simulink model "quadcopter_sim_1"  (R2023b)
settings: Solver=VariableStepAuto  StartTime=0.0  StopTime=10  RelTol=1e-3
libraries: simulink x2, mpclib x1, aerolibanimutils x1
settings Model: Creator=farhan  LastModifiedBy=farhan

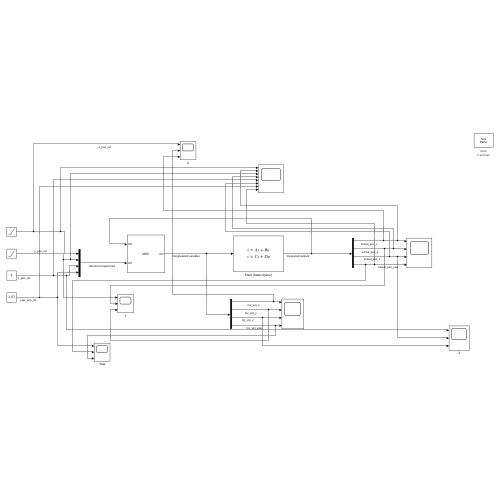
[thumbnail: Simulink's stored preview of the top-level diagram]
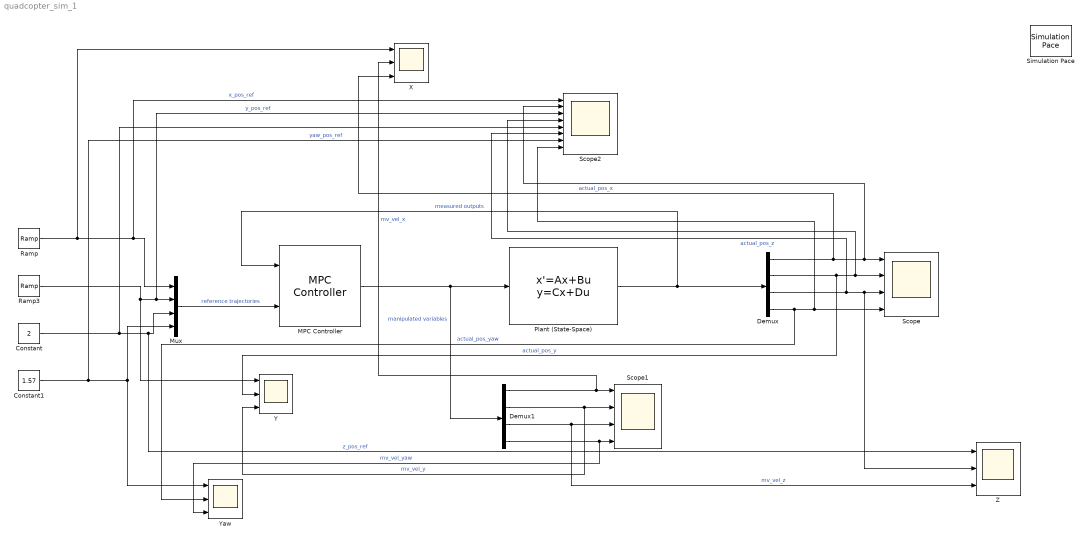
== system quadcopter_sim_1 ==
  Constant : Constant  Value=2
  Constant1 : Constant  Value=1.57
  Demux : Demux
  Demux1 : Demux
  MPC Controller : mpclib/MPC Controller  SCDEnableBlockLinearizationSpecification=on  mpcobj=mpc1  is_multiple=0  enable_value=0  return_u0=off  updateMPCinCallerWorkspace=on  md_inport=off  mv_inport=off  uref_inport=off  return_cost=off  return_mvseq=off  return_qpstatus=off  return_xseq=off  return_state=off  return_ovseq=off  state_inport=off  umin_inport=off  umax_inport=off  ymin_inport=off  ymax_inport=off  cc_inport=off  ywt_inport=off  uwt_inport=off  duwt_inport=off  rhoeps_inport=off  pm_inport=off  MaximumP=10  HorizonChoice=FixedHorizon  n_ts=0.1  n_p=20  n_mv=4  n_md=0  n_ud=0  n_mo=4  n_uo=0  BlockDataType=double  SampleTimeInherited=off  switch_inport=off
  Mux : Mux
  Plant (State-Space) : StateSpace  A=[0, 0, 0, 0; 0, 0, 0, 0; 0, 0, 0, 0; 0, 0, 0, 0]  B=[1, 0, 0, 0; 0, 1, 0, 0; 0, 0, 1, 0; 0, 0, 0, 1]  C=[1, 0, 0, 0; 0, 1, 0, 0; 0, 0, 1, 0; 0, 0, 0, 1]  D=[0, 0, 0, 0; 0, 0, 0, 0; 0, 0, 0, 0; 0, 0, 0, 0]  InitialCondition=[0, 0, 2, 1.57]  ContinuousStateAttributes='position'
  Ramp : simulink/Sources/Ramp  slope=0.3  start=0  InitialOutput=0
  Ramp3 : simulink/Sources/Ramp  slope=0.3  start=0  InitialOutput=0
  Scope : Scope  NumInputPorts=4
  Scope1 : Scope  NumInputPorts=4
  Scope2 : Scope  NumInputPorts=8
  Simulation Pace : aerolibanimutils/Simulation Pace  SimulationPace=1  SleepMode=Auto  OutputPaceError=off  SampleTime=1/30
  X : Scope  NumInputPorts=3
  Y : Scope  NumInputPorts=3
  Yaw : Scope  NumInputPorts=3
  Z : Scope  NumInputPorts=3
  wires:
  MPC Controller/1 -> Plant (State-Space)/1, Demux1/1  "manipulated variables"
  Plant (State-Space)/1 -> Demux/1, MPC Controller/1  "measured outputs"
  Mux/1 -> MPC Controller/2  "reference trajectories"
  Ramp3/1 -> Y/1, Scope2/3, Mux/2  "y_pos_ref"
  Constant/1 -> Z/1, Mux/3, Scope2/5  "z_pos_ref"
  Demux/1 -> X/3, Scope2/2, Scope/1  "actual_pos_x"
  Demux/2 -> Y/2, Scope2/4, Scope/2  "actual_pos_y"
  Demux/3 -> Scope2/6, Z/2, Scope/3  "actual_pos_z"
  Demux/4 -> Yaw/2, Scope2/8, Scope/4  "actual_pos_yaw"
  Demux1/4 -> Yaw/3, Scope1/4  "mv_vel_yaw"
  Demux1/3 -> Z/3, Scope1/3  "mv_vel_z"
  Demux1/2 -> Y/3, Scope1/2  "mv_vel_y"
  Demux1/1 -> Scope1/1, X/2  "mv_vel_x"
  Ramp/1 -> Mux/1, Scope2/1, X/1  "x_pos_ref"
  Constant1/1 -> Yaw/1, Mux/4, Scope2/7  "yaw_pos_ref"
